simulink model "topic2"  (R2019b)
settings: Solver=VariableStepAuto  StartTime=0.0  StopTime=0.09  RelTol=1e-3
libraries: powerlib x21, powerlib_meascontrol x8
settings Model: Creator=96547  LastModifiedBy=96547

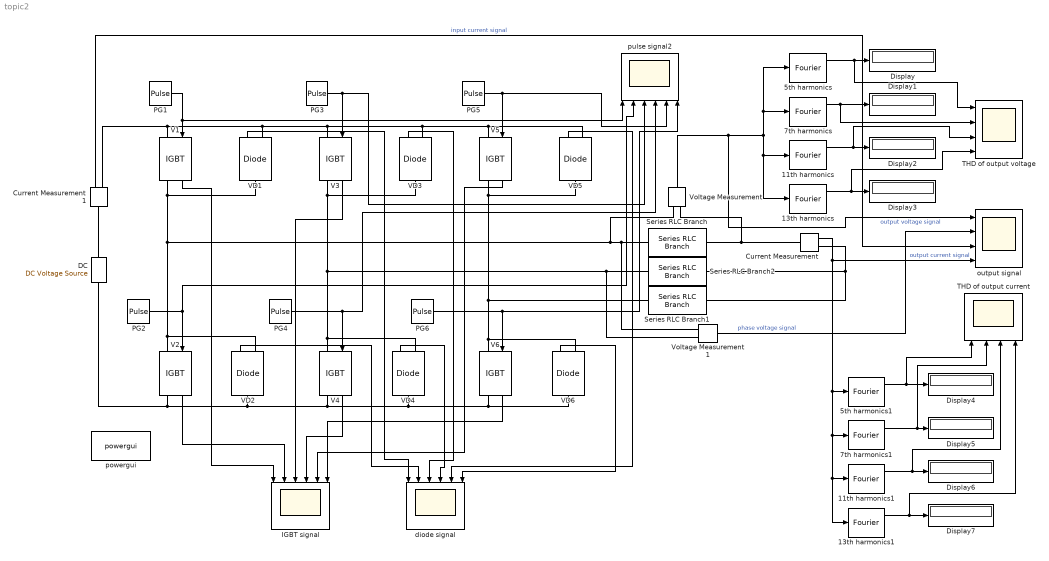
== system topic2 ==
  11th harmonics : powerlib_meascontrol/Measurements/Fourier  Freq=50  n=11  InInit=[0, 0]  Ts=0
      settings: SourceProductName=Simscape Electrical
  11th harmonics1 : powerlib_meascontrol/Measurements/Fourier  Freq=50  n=11  InInit=[0, 0]  Ts=0
      settings: SourceProductName=Simscape Electrical
  13th harmonics : powerlib_meascontrol/Measurements/Fourier  Freq=50  n=13  InInit=[0, 0]  Ts=0
      settings: SourceProductName=Simscape Electrical
  13th harmonics1 : powerlib_meascontrol/Measurements/Fourier  Freq=50  n=13  InInit=[0, 0]  Ts=0
      settings: SourceProductName=Simscape Electrical
  5th harmonics : powerlib_meascontrol/Measurements/Fourier  Freq=50  n=5  InInit=[0, 0]  Ts=0
      settings: SourceProductName=Simscape Electrical
  5th harmonics1 : powerlib_meascontrol/Measurements/Fourier  Freq=50  n=5  InInit=[0, 0]  Ts=0
      settings: SourceProductName=Simscape Electrical
  7th harmonics : powerlib_meascontrol/Measurements/Fourier  Freq=50  n=7  InInit=[0, 0]  Ts=0
      settings: SourceProductName=Simscape Electrical
  7th harmonics1 : powerlib_meascontrol/Measurements/Fourier  Freq=50  n=7  InInit=[0, 0]  Ts=0
      settings: SourceProductName=Simscape Electrical
  Current Measurement : powerlib/Measurements/Current Measurement  PhasorSimulation=off  OutputType=Complex  PSBequivalent=0
      settings: SourceProductName=Simscape Electrical
  Current Measurement1 : powerlib/Measurements/Current Measurement  PhasorSimulation=off  OutputType=Complex  PSBequivalent=0
      settings: SourceProductName=Simscape Electrical
  DC : powerlib/Electrical Sources/DC Voltage Source  Amplitude=400  Measurements=None
      settings: SourceProductName=Simscape Electrical
  Display{,1..7} (8 alike) : Display
  IGBT signal : Scope  NumInputPorts=6
  PG1 : DiscretePulseGenerator  PulseType=Time based  Period=0.02  PulseWidth=50
  PG2 : DiscretePulseGenerator  PulseType=Time based  Period=0.02  PulseWidth=50  PhaseDelay=0.01
  PG3 : DiscretePulseGenerator  PulseType=Time based  Period=0.02  PulseWidth=50  PhaseDelay=0.02*(1/3)
  PG4 : DiscretePulseGenerator  PulseType=Time based  Period=0.02  PulseWidth=50  PhaseDelay=0.01+0.02*(1/3)
  PG5 : DiscretePulseGenerator  PulseType=Time based  Period=0.02  PulseWidth=50  PhaseDelay=0.02*(2/3)
  PG6 : DiscretePulseGenerator  PulseType=Time based  Period=0.02  PulseWidth=50  PhaseDelay=0.01+0.02*(2/3)
  Series RLC Branch : powerlib/Elements/Series RLC Branch  LConnTagsString=__new0  RConnTagsString=__new0  BranchType=RL  Resistance=5  Inductance=0.01  SetiL0=off  InitialCurrent=0  Capacitance=1e-6  Setx0=off  InitialVoltage=0  Measurements=None
      settings: SourceProductName=Simscape Electrical
  Series RLC Branch1 : powerlib/Elements/Series RLC Branch  LConnTagsString=__new0  RConnTagsString=__new0  BranchType=RL  Resistance=5  Inductance=0.01  SetiL0=off  InitialCurrent=0  Capacitance=1e-6  Setx0=off  InitialVoltage=0  Measurements=None
      settings: SourceProductName=Simscape Electrical
  Series RLC Branch2 : powerlib/Elements/Series RLC Branch  LConnTagsString=__new0  RConnTagsString=__new0  BranchType=RL  Resistance=5  Inductance=0.01  SetiL0=off  InitialCurrent=0  Capacitance=1e-6  Setx0=off  InitialVoltage=0  Measurements=None
      settings: SourceProductName=Simscape Electrical
  THD of output current : Scope  NumInputPorts=4
  THD of output voltage : Scope  NumInputPorts=4
  V{1..6} (6 alike) : powerlib/Power Electronics/IGBT  Ron=0.001  Lon=0  Vf=1  Tf=1e-6  Tt=2e-6  IC=0  Rs=1e5  Cs=inf  Measurements=on
      settings: SourceProductName=Simscape Electrical
  VD{1..6} (6 alike) : powerlib/Power Electronics/Diode  Ron=0.001  Lon=0  Vf=0.8  IC=0  UseSnubber=0  Rs=500  Cs=250e-9  Measurements=on
      settings: SourceProductName=Simscape Electrical
  Voltage Measurement : powerlib/Measurements/Voltage Measurement  PhasorSimulation=off  OutputType=Complex  PSBequivalent=0
      settings: SourceProductName=Simscape Electrical
  Voltage Measurement1 : powerlib/Measurements/Voltage Measurement  PhasorSimulation=off  OutputType=Complex  PSBequivalent=0
      settings: SourceProductName=Simscape Electrical
  diode signal : Scope  NumInputPorts=6
  output signal : Scope  NumInputPorts=4
  powergui : powerlib/powergui  Priority=1  SimulationMode=Continuous  SampleTime=50e-6  frequency=60  Iterations=50  frequencyindice=0  Pbase=100e6  ErrMax=1e-4  UnitsV=kV  UnitsW=MW  buscounter=0  FunctionMessages=off  echomessages=off  EnableUseOfTLC=off  CurrentSourceSwitches=off  DisableSnubberDevices=off  DisableRonSwitches=off  DisableVfSwitches=off  DisplayEquations=off  AutomaticDiscreteSolvers=off  SolverType=Tustin/Backward Euler (TBE)  Interpol=off  ExternalGateDelay=off  methode=off  Ts=100  x0status=blocks  SPID=on  SwTol=0  HookPort=off  NonlinearTolerance=1e-4  nMaxIteration=100  ContinueOnMaxIteration=off  RestoreLinks=warning  ResistiveCurrentMeasurement=off  Frange=[0:2:500]  Ylog=off  Xlog=on  ShowGrid=off  save=off  variable=ZData  structure=0  ZoomFFT=off  StartTime=0.0  cycles=1  DisplayStyle=1  fundamental=60  FreqAxis=off  MaxFrequency=1000  frequencyindicesteady=1  RmsSteady=1  display=off
      settings: SourceProductName=Simscape Electrical
  pulse signal2 : Scope  NumInputPorts=6
  wires:
  PG1/1 -> pulse signal2/1, V1/1
  VD1/1 -> diode signal/1
  VD2/1 -> diode signal/2
  VD3/1 -> diode signal/3
  VD4/1 -> diode signal/4
  VD5/1 -> diode signal/5
  VD6/1 -> diode signal/6
  V1/1 -> IGBT signal/1
  V2/1 -> IGBT signal/2
  V3/1 -> IGBT signal/3
  V4/1 -> IGBT signal/4
  V5/1 -> IGBT signal/5
  V6/1 -> IGBT signal/6
  PG3/1 -> pulse signal2/3, V3/1
  PG5/1 -> pulse signal2/5, V5/1
  Voltage Measurement/1 -> output signal/1, 13th harmonics/1, 11th harmonics/1, 5th harmonics/1, 7th harmonics/1  "output voltage signal"
  5th harmonics/1 -> THD of output voltage/1, Display/1
  7th harmonics/1 -> THD of output voltage/2, Display1/1
  11th harmonics/1 -> THD of output voltage/3, Display2/1
  13th harmonics/1 -> THD of output voltage/4, Display3/1
  PG2/1 -> pulse signal2/2, V2/1
  PG4/1 -> pulse signal2/4, V4/1
  PG6/1 -> pulse signal2/6, V6/1
  13th harmonics1/1 -> THD of output current/4, Display7/1
  11th harmonics1/1 -> THD of output current/3, Display6/1
  7th harmonics1/1 -> THD of output current/2, Display5/1
  5th harmonics1/1 -> THD of output current/1, Display4/1
  Current Measurement/1 -> 5th harmonics1/1, 7th harmonics1/1, 11th harmonics1/1, 13th harmonics1/1, output signal/4  "output current signal"
  Current Measurement1/1 -> output signal/3  "input current signal"
  Voltage Measurement1/1 -> output signal/2  "phase voltage signal"
  connections:
  V1/LConn1 -- VD3/RConn1 -- VD5/RConn1 -- V5/LConn1 -- V3/LConn1 -- VD1/RConn1 -- Current Measurement1/RConn1
  DC/LConn1 -- V2/RConn1 -- VD6/LConn1 -- V6/RConn1 -- VD4/LConn1 -- V4/RConn1 -- VD2/LConn1
  V2/LConn1 -- VD2/RConn1 -- Voltage Measurement/LConn1 -- Voltage Measurement1/LConn1 -- Series RLC Branch/LConn1 -- VD1/LConn1 -- V1/RConn1
  V6/LConn1 -- VD6/RConn1 -- VD5/LConn1 -- V5/RConn1 -- Series RLC Branch1/LConn1
  V4/LConn1 -- VD4/RConn1 -- Voltage Measurement1/LConn2 -- Series RLC Branch2/LConn1 -- VD3/LConn1 -- V3/RConn1
  Series RLC Branch1/RConn1 -- Series RLC Branch2/RConn1 -- Current Measurement/RConn1
  Current Measurement/LConn1 -- Voltage Measurement/LConn2 -- Series RLC Branch/RConn1
  DC/RConn1 -- Current Measurement1/LConn1
